simulink subsystem "Mk3SerialImpairments"  (R2025a)
settings: Solver=VariableStepAuto  StartTime=0.0  StopTime=10.0  RelTol=1e-3
undefined symbols (not defined in the file): MCU_Ts
libraries: arsenal x1
settings Model: DataDictionary=neck_mk3.sldd  EnableAccessToBaseWorkspace=off  Creator=upattacini  LastModifiedBy=upattacini

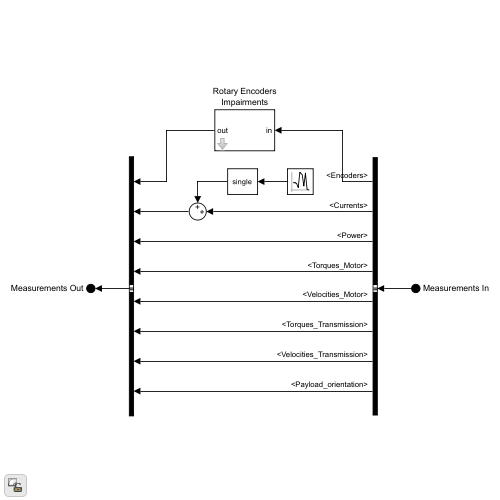
[thumbnail: Simulink's stored preview of the top-level diagram]
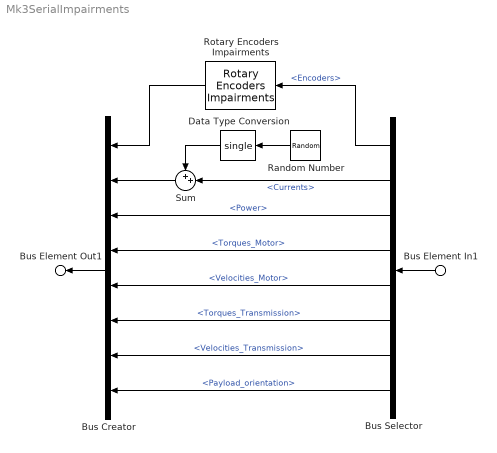
== system Mk3SerialImpairments ==
  Bus Element In1 : Inport  PortName=Measurements In
  Bus Creator : BusCreator  Inputs=8  OutDataTypeStr=Bus: Data_Measurements  NonVirtualBus=on
      settings: InheritFromInputs=off
  Bus Selector : BusSelector  OutputSignals=Encoders,Currents,Power,Torques_Motor,Velocities_Motor,Torques_Transmission,Velocities_Transmission,Payload_orientation
  Data Type Conversion : DataTypeConversion  OutDataTypeStr=single  SaturateOnIntegerOverflow=off  RndMeth=Floor
  Random Number : RandomNumber  Variance=0  SampleTime=MCU_Ts
  Rotary Encoders Impairments : arsenal/Sensing/Rotary Encoders Impairments  bit_resolution=14  bit_noise=2  seed=0  Ts=MCU_Ts
  Sum : Sum  Inputs=++|
  Bus Element Out1 : Outport  PortName=Measurements Out
  wires:
  Bus Element In1/1 -> Bus Selector/1
  Bus Creator/1 -> Bus Element Out1/1
  Bus Selector/3 -> Bus Creator/3  "<Power>"
  Bus Selector/4 -> Bus Creator/4  "<Torques_Motor>"
  Bus Selector/5 -> Bus Creator/5  "<Velocities_Motor>"
  Bus Selector/6 -> Bus Creator/6  "<Torques_Transmission>"
  Bus Selector/7 -> Bus Creator/7  "<Velocities_Transmission>"
  Bus Selector/8 -> Bus Creator/8  "<Payload_orientation>"
  Bus Selector/1 -> Rotary Encoders Impairments/1  "<Encoders>"
  Rotary Encoders Impairments/1 -> Bus Creator/1
  Sum/1 -> Bus Creator/2
  Bus Selector/2 -> Sum/2  "<Currents>"
  Random Number/1 -> Data Type Conversion/1
  Data Type Conversion/1 -> Sum/1
